simulink model "lab4pt2k2"  (Simulink 8.0)
settings: Solver=ode1  StartTime=0.0  StopTime=10  FixedStep=0.002  RelTol=1e-3
libraries: simulink_extras x1
settings Model: Creator=vukovic8  LastModifiedBy=vukovic8  ExtModeTrigDuration=5000
settings SolverCC: PositivePriorityOrder=on
settings RTWCC: SystemTargetFile=quarc_win64.tlc  TemplateMakefile=quarc_default_tmf  Description=QUARC Win64 Target  ProcessScript=quarc_win64_make_rtw_hook
settings STFCustomTargetCC: TargetPreCompLibLocation=C:\PROGRA~3\QUARC\lib\2012b\win64\release  CodeReplacementLibrary=ANSI_C  GeneratePreprocessorConditionals=Disable all  CombineOutputUpdateFcns=on  GRTInterface=off  SystemTargetFile=quarc_win64.tlc
settings GRTTargetCC: TargetPreCompLibLocation=C:\PROGRA~3\QUARC\lib\2012b\win64\release  ParMdlRefBuildCompliant=off  CompOptLevelCompliant=off  ConcurrentExecutionCompliant=off  MatFileLogging=off  ExtMode=on  ExtModeMexFile=quarc_comm

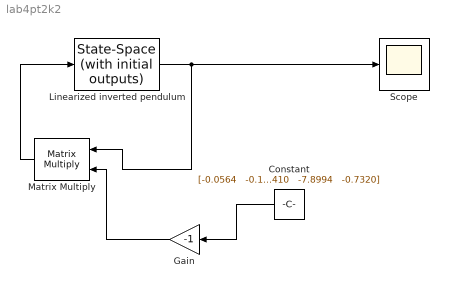
== system lab4pt2k2 ==
  Constant : Constant  Value="[-0.0564   -0.1410   -7.8994   -0.7320]"
  Gain : Gain  Gain=-1
  Linearized inverted pendulum : simulink_extras/Additional Linear/State-Space (with initial outputs)  A=[0,1,0,0; 0,0,-4.5138,0; 0,0,0,1; 0,0,47.1744,0]  B=[0; 2.1978; 0; -7.2535]  C=eye(4)  D=[0;0;0;0]  U0=1  Y0=[0; 0; 0.035; 0.01]
  Matrix Multiply : Product  Multiplication=Matrix(*)
  Scope : Scope
      settings: ShowLegends=on
  wires:
  Linearized inverted pendulum/1 -> Scope/1, Matrix Multiply/1
  Matrix Multiply/1 -> Linearized inverted pendulum/1
  Constant/1 -> Gain/1
  Gain/1 -> Matrix Multiply/2
